simulink model "myexp7_2"  (R2022a)
settings: Solver=VariableStepAuto  StartTime=0.0  StopTime=10  RelTol=1e-3
libraries: commchan3 x1, commrandsrc3 x1, commsink2 x1, commfilt2 x1, dspfdesign x1, dspstat3 x1, dspsigops x1
settings Model: Creator=惠普  LastModifiedBy=惠普

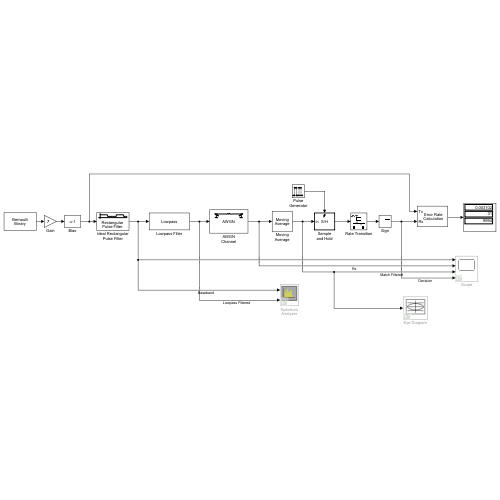
[thumbnail: Simulink's stored preview of the top-level diagram]
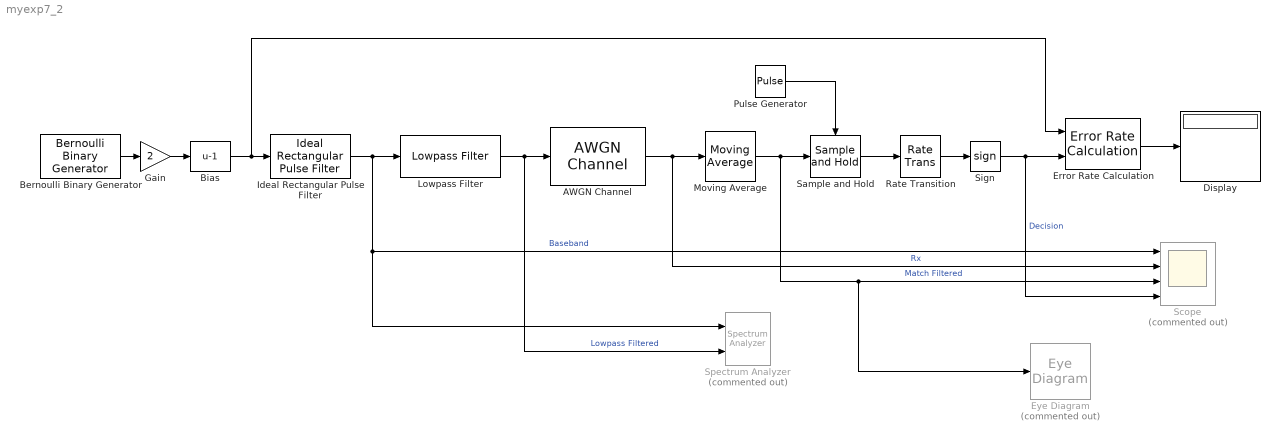
== system myexp7_2 ==
  AWGN Channel : commchan3/AWGN Channel  InputProcessing=Columns as channels (frame based)  seed=137  noiseMode="Signal to noise ratio  (Es/No)"  EbNodB=10  EsNodB=10  SNRdB=10  bitsPerSym=1  Ps=1  Tsym=1e-3  variance=1
  Bernoulli Binary Generator : commrandsrc3/Bernoulli Binary Generator  ProbabilityOfZero=0.5  SeedSource=Auto  Seed=0  SampleTime=1e-3  SamplesPerFrame=1  OutputDataType=double  SimulateUsing=Interpreted execution
  Bias : Bias  Bias=-1  SaturateOnIntegerOverflow=off
  Display : Display
  Error Rate Calculation : commsink2/Error Rate Calculation  N=7  st_delay=0  cp_mode=Entire frame  subframe=[]  PMode=Port  WsName=ErrorVec  RsMode2=off  stop=off  numErr=100  maxBits=1e6
  Eye Diagram : EyeDiagram  Commented=on
  Gain : Gain  Gain=2
  Ideal Rectangular Pulse Filter : commfilt2/Ideal Rectangular Pulse Filter  pulseLen=100  pulseDelay=0  InputProcessing=Columns as channels (frame based)  RateOptions=Allow multirate processing  sampMode=Mute  normCheck=off  normMode=Sum of samples  filterGain=1  saveAsFlag=0  roundingMode=Floor  overflowMode=off  firstCoeffDataTypeStr=Inherit: Same word length as input  firstCoeffMin=[]  firstCoeffMax=[]  firstCoeffLastDataTypeStr=Inherit: Same word length as input  outputDataTypeStr=Inherit: Same as accumulator  outputMin=[]  outputMax=[]  outputLastDataTypeStr=Inherit: Same as accumulator
      settings: SourceProductBaseCode=CM
  Lowpass Filter : dspfdesign/Lowpass Filter  FilterType=FIR  DesignForMinimumOrder=on  FilterOrder=50  PassbandFrequency=0.4e3  StopbandFrequency=0.6e3  PassbandRipple=0.1  StopbandAttenuation=40  InheritSampleRate=off  SampleRate=100e3  SimulateUsing=Interpreted execution  roundingMode=Floor  coeffsDataTypeStr=fixdt(1,16)
  Moving Average : dspstat3/Moving Average  Method=Sliding window  ForgettingFactorPort=off  SpecifyWindowLength=on  WindowLength=100  ForgettingFactor=0.9  SimulateUsing=Code generation
  Pulse Generator : DiscretePulseGenerator  Period=100  PhaseDelay=28  SampleTime=10e-6
  Rate Transition : RateTransition  OutPortSampleTime=1e-3
  Sample and Hold : dspsigops/Sample and Hold  trig=Rising edge  initCond=0  latchinput=off
  Scope : Scope  Commented=on  NumInputPorts=4
  Sign : Signum
  Spectrum Analyzer : SpectrumAnalyzer  Commented=on  NumInputPorts=2
  wires:
  Bernoulli Binary Generator/1 -> Gain/1
  Gain/1 -> Bias/1
  Bias/1 -> Error Rate Calculation/1, Ideal Rectangular Pulse Filter/1
  AWGN Channel/1 -> Scope/2, Moving Average/1  "Rx"
  Moving Average/1 -> Eye Diagram/1, Scope/3, Sample and Hold/1  "Match Filtered"
  Pulse Generator/1 -> Sample and Hold/Trigger
  Sample and Hold/1 -> Rate Transition/1
  Rate Transition/1 -> Sign/1
  Sign/1 -> Scope/4, Error Rate Calculation/2  "Decision"
  Error Rate Calculation/1 -> Display/1
  Ideal Rectangular Pulse Filter/1 -> Scope/1, Spectrum Analyzer/1, Lowpass Filter/1  "Baseband"
  Lowpass Filter/1 -> Spectrum Analyzer/2, AWGN Channel/1  "Lowpass Filtered"
